simulink model "Dyn_Nonlinear_Forcefour"  (R2021a)
settings: Solver=VariableStepAuto  StartTime=0.0  StopTime=5  FixedStep=0.048  MaxStep=0.048  RelTol=1e-5
settings Model: Creator=zahra  LastModifiedBy=Dell 5520
settings SolverCC: AlgebraicLoopSolver=TrustRegion
settings DataIOCC: ReturnWorkspaceOutputs=off
settings DebuggingCC: ArithmeticOperatorsInVariantConditions=warning
settings SFSimCC: CustomCodeUndefinedFunction=UseInterfaceOnly
settings CodeAppCC: StateflowObjectComments=on

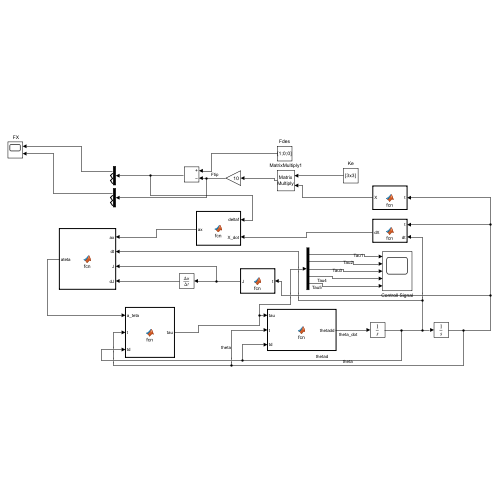
[thumbnail: Simulink's stored preview of the top-level diagram]
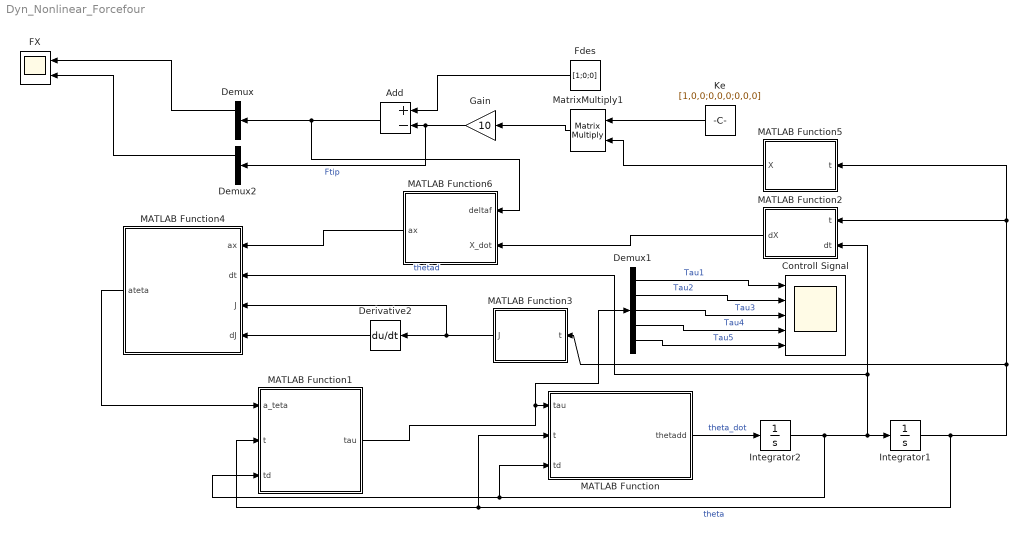
== system Dyn_Nonlinear_Forcefour ==
  " FX" : Scope  NumInputPorts=2
  Add : Sum  Inputs=+-
  Controll Signal : Scope  NumInputPorts=5
  Demux : Demux  Outputs=3
  Demux1 : Demux  Outputs=5
  Demux2 : Demux  Outputs=3
  Derivative2 : Derivative
  Fdes : Constant  Value=[1;0;0]
  Gain : Gain  Gain=10
  Integrator1 : Integrator  InitialCondition=[0;0;0;0;0]
  Integrator2 : Integrator  InitialCondition=[0;0;0;0;0]
  Ke : Constant  Value=[1,0,0;0,0,0;0,0,0]
  MATLAB Function : MATLAB Function  TreatAsAtomicUnit=on
  MATLAB Function1 : MATLAB Function  TreatAsAtomicUnit=on
  MATLAB Function2 : MATLAB Function  TreatAsAtomicUnit=on
  MATLAB Function3 : MATLAB Function  TreatAsAtomicUnit=on
  MATLAB Function4 : MATLAB Function  TreatAsAtomicUnit=on
  MATLAB Function5 : MATLAB Function  TreatAsAtomicUnit=on
  MATLAB Function6 : MATLAB Function  TreatAsAtomicUnit=on
  MatrixMultiply1 : Product  Multiplication=Matrix(*)
  wires:
  MATLAB Function/1(thetadd) -> Integrator2/1  "theta_dot"
  Integrator1/1 -> MATLAB Function5/1(t), MATLAB Function2/1(t), MATLAB Function3/1(t), MATLAB Function/2(t), MATLAB Function1/2(t)  "theta"
  Integrator2/1 -> MATLAB Function2/2(dt), MATLAB Function4/2(dt), Integrator1/1, MATLAB Function/3(td), MATLAB Function1/3(td)  "thetad"
  MATLAB Function1/1(tau) -> Demux1/1, MATLAB Function/1(tau)
  MATLAB Function3/1(J) -> MATLAB Function4/3(J), Derivative2/1
  Derivative2/1 -> MATLAB Function4/4(dJ)
  MATLAB Function6/1(ax) -> MATLAB Function4/1(ax)
  MATLAB Function4/1(ateta) -> MATLAB Function1/1(a_teta)
  MATLAB Function5/1(X) -> MatrixMultiply1/2
  MATLAB Function2/1(dX) -> MATLAB Function6/2(X_dot)
  Ke/1 -> MatrixMultiply1/1
  MatrixMultiply1/1 -> Gain/1
  Add/1 -> MATLAB Function6/1(deltaf), Demux/1
  Fdes/1 -> Add/1
  Demux/1 -> " FX"/1
  Gain/1 -> Demux2/1, Add/2  "Ftip"
  Demux1/4 -> Controll Signal/4  "Tau4"
  Demux1/5 -> Controll Signal/5  "Tau5"
  Demux1/1 -> Controll Signal/1  "Tau1"
  Demux1/2 -> Controll Signal/2  "Tau2"
  Demux1/3 -> Controll Signal/3  "Tau3"
  Demux2/1 -> " FX"/2

== matlab function Dyn_Nonlinear_Forcefour/MATLAB Function2 ==
  data: t input; dX output; dt input
function dX  = fcn(t,dt)
theta1 = t(1); theta2 = t(2); theta3 = t(3); 
theta4 = t(4); theta5 = t(5); 


T01 = [cos(theta1),0,sin(theta1),0;sin(theta1),0,-cos(theta1),0;0,1,0,0;0,0,0,1];
T12 = [cos(theta2),-sin(theta2),0,0.50*cos(theta2);sin(theta2),cos(theta2),0,0.50*sin(theta2);0,0,1,0;0,0,0,1];
T23 = [cos(theta3),-sin(theta3),0,0.50*cos(theta3);sin(theta3),cos(theta3),0,0.50*sin(theta3);0,0,1,0;0,0,0,1];
T34 = [cos(theta4),0,-sin(theta4),0;sin(theta4),0,cos(theta4),0;0,-1,0,0;0,0,0,1];
T45 = [cos(theta5),-sin(theta5),0,0;sin(theta5),cos(theta5),0,0;0,0,1,0.15;0,0,0,1];

T02 = T01 * T12 ;
T03 = T01 * T12 * T23 ; 
T04 = T01 * T12 * T23 * T34 ;
T0e=  T01 * T12 * T23 * T34 * T45 ;

z1 = T01(1:3, 3);
z2 = T02(1:3, 3);
z3 = T03(1:3, 3);
z4 = T04(1:3, 3);
z5 = T0e(1:3, 3);

o1 = T01(1:3, 4);
o2 = T02(1:3, 4);
o3 = T03(1:3, 4);
o4 = T04(1:3, 4);
o5 = T0e(1:3, 4);

J1 = [cross(z1, (o5 - o1))];
J2 = [cross(z2, (o5 - o2))];
J3 = [cross(z3, (o5 - o3))];
J4 = [cross(z4, (o5 - o4))];
J5 = [cross(z5, (o5 - o5))];
J_alternative_V = [J1 J2 J3 J4 J5];

J=J_alternative_V;

dX=J*dt;
return;

== matlab function Dyn_Nonlinear_Forcefour/MATLAB Function1 ==
  data: a_teta input; tau output; t input; td input
function tau  = fcn(a_teta, t, td)

theta1 = t(1); theta2 = t(2); theta3 = t(3); 
theta4 = t(4); theta5 = t(5);  

thetad1 = td(1); thetad2 = td(2); thetad3 = td(3);
thetad4 = td(4); thetad5 = td(5); 

M=zeros(5);
M(1,1) = 1.1807*cos(theta3) - 0.9672*cos(theta4) - 0.7031*sin(theta3) - 1.7889*sin(theta4) - 0.9672*cos(theta3)*cos(theta4) - 1.7889*cos(theta3)*sin(theta4) - 1.7889*cos(theta4)*sin(theta3) - 1.84*cos(theta5)*sin(theta5) + 0.9672*sin(theta3)*sin(theta4) - 1.17*cos(theta5)^2 + 11.017252 ;
M(1,2) = 0.59035*cos(theta3) - 0.9672*cos(theta4) - 0.35155*sin(theta3) - 1.7889*sin(theta4) - 0.4836*cos(theta3)*cos(theta4) - 0.89445*cos(theta3)*sin(theta4) - 0.89445*cos(theta4)*sin(theta3) - 1.84*cos(theta5)*sin(theta5) + 0.4836*sin(theta3)*sin(theta4) - 1.17*cos(theta5)^2 + 10.020592 ;
M(1,3) = 0.4836*sin(theta3)*sin(theta4) - 0.4836*cos(theta4) - 0.35155*sin(theta3) - 0.89445*sin(theta4) - 0.4836*cos(theta3)*cos(theta4) - 0.89445*cos(theta3)*sin(theta4) - 0.89445*cos(theta4)*sin(theta3) - 1.84*cos(theta5)*sin(theta5) - 0.16465*cos(theta3) - 1.17*cos(theta5)^2 + 9.175155 ;
M(1,4) = 0.98*sin(theta5) - 0.8928*sin(theta4) - 1.67*cos(theta5) - 0.8928*cos(theta3)*sin(theta4) - 0.8928*cos(theta4)*sin(theta3) + 0.008464 ;
M(1,5) = 0.98*sin(theta5) - 1.67*cos(theta5) ;
M(2,1) = 0.59035*cos(theta3) - 0.9672*cos(theta4) - 0.35155*sin(theta3) - 1.7889*sin(theta4) - 0.4836*cos(theta3)*cos(theta4) - 0.89445*cos(theta3)*sin(theta4) - 0.89445*cos(theta4)*sin(theta3) - 1.84*cos(theta5)*sin(theta5) + 0.4836*sin(theta3)*sin(theta4) - 1.17*cos(theta5)^2 + 10.020592 ;
M(2,2) = 10.133642 - 1.7889*sin(theta4) - 1.84*cos(theta5)*sin(theta5) - 1.17*cos(theta5)^2 - 0.9672*cos(theta4) ;
M(2,3) = 9.175155 - 0.89445*sin(theta4) - 1.84*cos(theta5)*sin(theta5) - 1.17*cos(theta5)^2 - 0.4836*cos(theta4) ;
M(2,4) = 0.98*sin(theta5) - 0.8928*sin(theta4) - 1.67*cos(theta5) + 0.008464 ;
M(2,5) = 0.98*sin(theta5) - 1.67*cos(theta5) ;
M(3,1) = 0.4836*sin(theta3)*sin(theta4) - 0.4836*cos(theta4) - 0.35155*sin(theta3) - 0.89445*sin(theta4) - 0.4836*cos(theta3)*cos(theta4) - 0.89445*cos(theta3)*sin(theta4) - 0.89445*cos(theta4)*sin(theta3) - 1.84*cos(theta5)*sin(theta5) - 0.16465*cos(theta3) - 1.17*cos(theta5)^2 + 9.175155 ;
M(3,2) = 9.175155 - 0.89445*sin(theta4) - 1.84*cos(theta5)*sin(theta5) - 1.17*cos(theta5)^2 - 0.4836*cos(theta4) ;
M(3,3) = 9.339805 - 1.17*cos(theta5)^2 - 1.84*cos(theta5)*sin(theta5) ;
M(3,4) = 0.98*sin(theta5) - 1.67*cos(theta5) + 0.008464 ;
M(3,5) = 0.98*sin(theta5) - 1.67*cos(theta5) ;
M(4,1) = 0.98*sin(theta5) - 0.8928*sin(theta4) - 1.67*cos(theta5) - 0.8928*cos(theta3)*sin(theta4) - 0.8928*cos(theta4)*sin(theta3) + 0.008464 ;
M(4,2) = 0.98*sin(theta5) - 0.8928*sin(theta4) - 1.67*cos(theta5) + 0.008464 ;
M(4,3) = 0.98*sin(theta5) - 1.67*cos(theta5) + 0.008464 ;
M(4,4) = 6.81712 ;
M(4,5) = 2.3 ;
M(5,1) = 0.98*sin(theta5) - 1.67*cos(theta5) ;
M(5,2) = 0.98*sin(theta5) - 1.67*cos(theta5) ;
M(5,3) = 0.98*sin(theta5) - 1.67*cos(theta5) ;
M(5,4) = 2.3 ;
M(5,5) = 2.3 ;


C=zeros(5);
C(1,1) = 0.92*thetad5 - 1.84*thetad5*cos(theta5)^2 - 0.35155*thetad3*cos(theta3) - 0.89445*thetad4*cos(theta4) - 0.59035*thetad3*sin(theta3) + 0.4836*thetad4*sin(theta4) - 0.89445*thetad3*cos(theta3)*cos(theta4) - 0.89445*thetad4*cos(theta3)*cos(theta4) + 0.4836*thetad3*cos(theta3)*sin(theta4) + 0.4836*thetad3*cos(theta4)*sin(theta3) + 0.4836*thetad4*cos(theta3)*sin(theta4) + 0.4836*thetad4*cos(theta4)*sin(theta3) + 1.17*thetad5*cos(theta5)*sin(theta5) + 0.89445*thetad3*sin(theta3)*sin(theta4) + 0.89445*thetad4*sin(theta3)*sin(theta4) ;
C(1,2) = 0.92*thetad5 - 1.84*thetad5*cos(theta5)^2 - 0.175775*thetad3*cos(theta3) - 0.89445*thetad4*cos(theta4) - 0.295175*thetad3*sin(theta3) + 0.4836*thetad4*sin(theta4) - 0.447225*thetad3*cos(theta3)*cos(theta4) - 0.447225*thetad4*cos(theta3)*cos(theta4) + 0.2418*thetad3*cos(theta3)*sin(theta4) + 0.2418*thetad3*cos(theta4)*sin(theta3) + 0.2418*thetad4*cos(theta3)*sin(theta4) + 0.2418*thetad4*cos(theta4)*sin(theta3) + 1.17*thetad5*cos(theta5)*sin(theta5) + 0.447225*thetad3*sin(theta3)*sin(theta4) + 0.447225*thetad4*sin(theta3)*sin(theta4) ;
C(1,3) = 0.92*thetad5 - 1.84*thetad5*cos(theta5)^2 - 0.35155*thetad1*cos(theta3) - 0.175775*thetad2*cos(theta3) - 0.35155*thetad3*cos(theta3) - 0.447225*thetad4*cos(theta4) - 0.59035*thetad1*sin(theta3) - 0.295175*thetad2*sin(theta3) + 0.16465*thetad3*sin(theta3) + 0.2418*thetad4*sin(theta4) - 0.89445*thetad1*cos(theta3)*cos(theta4) - 0.447225*thetad2*cos(theta3)*cos(theta4) - 0.89445*thetad3*cos(theta3)*cos(theta4) - 0.893625*thetad4*cos(theta3)*cos(theta4) + 0.4836*thetad1*cos(theta3)*sin(theta4) + 0.4836*thetad1*cos(theta4)*sin(theta3) + 0.2418*thetad2*cos(theta3)*sin(theta4) + 0.2418*thetad2*cos(theta4)*sin(theta3) + 0.4836*thetad3*cos(theta3)*sin(theta4) + 0.4836*thetad3*cos(theta4)*sin(theta3) + 0.2418*thetad4*cos(theta3)*sin(theta4) + 0.2418*thetad4*cos(theta4)*sin(theta3) + 1.17*thetad5*cos(theta5)*sin(theta5) + 0.89445*thetad1*sin(theta3)*sin(theta4) + 0.447225*thetad2*sin(theta3)*sin(theta4) + 0.89445*thetad3*sin(theta3)*sin(theta4) + 0.893625*thetad4*sin(theta3)*sin(theta4) ;
C(1,4) = 0.49*thetad5*cos(theta5) - 0.89445*thetad2*cos(theta4) - 0.447225*thetad3*cos(theta4) - 0.8928*thetad4*cos(theta4) - 0.89445*thetad1*cos(theta4) + 0.4836*thetad1*sin(theta4) + 0.4836*thetad2*sin(theta4) + 0.2418*thetad3*sin(theta4) + 0.835*thetad5*sin(theta5) - 0.89445*thetad1*cos(theta3)*cos(theta4) - 0.447225*thetad2*cos(theta3)*cos(theta4) - 0.893625*thetad3*cos(theta3)*cos(theta4) - 0.8928*thetad4*cos(theta3)*cos(theta4) + 0.4836*thetad1*cos(theta3)*sin(theta4) + 0.4836*thetad1*cos(theta4)*sin(theta3) + 0.2418*thetad2*cos(theta3)*sin(theta4) + 0.2418*thetad2*cos(theta4)*sin(theta3) + 0.2418*thetad3*cos(theta3)*sin(theta4) + 0.2418*thetad3*cos(theta4)*sin(theta3) + 0.89445*thetad1*sin(theta3)*sin(theta4) + 0.447225*thetad2*sin(theta3)*sin(theta4) + 0.893625*thetad3*sin(theta3)*sin(theta4) + 0.8928*thetad4*sin(theta3)*sin(theta4) ;
C(1,5) = 0.92*thetad1 + 0.92*thetad2 + 0.92*thetad3 - 1.84*thetad1*cos(theta5)^2 - 1.84*thetad2*cos(theta5)^2 - 1.84*thetad3*cos(theta5)^2 + 0.49*thetad4*cos(theta5) + 0.98*thetad5*cos(theta5) + 0.835*thetad4*sin(theta5) + 1.67*thetad5*sin(theta5) + 1.17*thetad1*cos(theta5)*sin(theta5) + 1.17*thetad2*cos(theta5)*sin(theta5) + 1.17*thetad3*cos(theta5)*sin(theta5) ;
C(2,1) = 0.92*thetad5 - 1.84*thetad5*cos(theta5)^2 - 0.175775*thetad3*cos(theta3) - 0.89445*thetad4*cos(theta4) - 0.295175*thetad3*sin(theta3) + 0.4836*thetad4*sin(theta4) - 0.447225*thetad3*cos(theta3)*cos(theta4) - 0.447225*thetad4*cos(theta3)*cos(theta4) + 0.2418*thetad3*cos(theta3)*sin(theta4) + 0.2418*thetad3*cos(theta4)*sin(theta3) + 0.2418*thetad4*cos(theta3)*sin(theta4) + 0.2418*thetad4*cos(theta4)*sin(theta3) + 1.17*thetad5*cos(theta5)*sin(theta5) + 0.447225*thetad3*sin(theta3)*sin(theta4) + 0.447225*thetad4*sin(theta3)*sin(theta4) ;
C(2,2) = 0.92*thetad5 - 1.84*thetad5*cos(theta5)^2 - 0.89445*thetad4*cos(theta4) + 0.4836*thetad4*sin(theta4) + 1.17*thetad5*cos(theta5)*sin(theta5) ;
C(2,3) = 0.92*thetad5 - 1.84*thetad5*cos(theta5)^2 - 0.175775*thetad1*cos(theta3) - 0.447225*thetad4*cos(theta4) - 0.295175*thetad1*sin(theta3) + 0.2418*thetad4*sin(theta4) - 0.447225*thetad1*cos(theta3)*cos(theta4) + 0.2418*thetad1*cos(theta3)*sin(theta4) + 0.2418*thetad1*cos(theta4)*sin(theta3) + 1.17*thetad5*cos(theta5)*sin(theta5) + 0.447225*thetad1*sin(theta3)*sin(theta4) ;
C(2,4) = 0.49*thetad5*cos(theta5) - 0.89445*thetad2*cos(theta4) - 0.447225*thetad3*cos(theta4) - 0.8928*thetad4*cos(theta4) - 0.89445*thetad1*cos(theta4) + 0.4836*thetad1*sin(theta4) + 0.4836*thetad2*sin(theta4) + 0.2418*thetad3*sin(theta4) + 0.835*thetad5*sin(theta5) - 0.447225*thetad1*cos(theta3)*cos(theta4) + 0.2418*thetad1*cos(theta3)*sin(theta4) + 0.2418*thetad1*cos(theta4)*sin(theta3) + 0.447225*thetad1*sin(theta3)*sin(theta4) ;
C(2,5) = 0.92*thetad1 + 0.92*thetad2 + 0.92*thetad3 - 1.84*thetad1*cos(theta5)^2 - 1.84*thetad2*cos(theta5)^2 - 1.84*thetad3*cos(theta5)^2 + 0.49*thetad4*cos(theta5) + 0.98*thetad5*cos(theta5) + 0.835*thetad4*sin(theta5) + 1.67*thetad5*sin(theta5) + 1.17*thetad1*cos(theta5)*sin(theta5) + 1.17*thetad2*cos(theta5)*sin(theta5) + 1.17*thetad3*cos(theta5)*sin(theta5) ;
C(3,1) = 0.92*thetad5 - 1.84*thetad5*cos(theta5)^2 + 0.35155*thetad1*cos(theta3) + 0.175775*thetad2*cos(theta3) - 0.447225*thetad4*cos(theta4) + 0.59035*thetad1*sin(theta3) + 0.295175*thetad2*sin(theta3) + 0.2418*thetad4*sin(theta4) + 0.89445*thetad1*cos(theta3)*cos(theta4) + 0.447225*thetad2*cos(theta3)*cos(theta4) - 0.000825*thetad4*cos(theta3)*cos(theta4) - 0.4836*thetad1*cos(theta3)*sin(theta4) - 0.4836*thetad1*cos(theta4)*sin(theta3) - 0.2418*thetad2*cos(theta3)*sin(theta4) - 0.2418*thetad2*cos(theta4)*sin(theta3) + 0.2418*thetad4*cos(theta3)*sin(theta4) + 0.2418*thetad4*cos(theta4)*sin(theta3) + 1.17*thetad5*cos(theta5)*sin(theta5) - 0.89445*thetad1*sin(theta3)*sin(theta4) - 0.447225*thetad2*sin(theta3)*sin(theta4) + 0.000825*thetad4*sin(theta3)*sin(theta4) ;
C(3,2) = 0.92*thetad5 - 1.84*thetad5*cos(theta5)^2 + 0.175775*thetad1*cos(theta3) - 0.447225*thetad4*cos(theta4) + 0.295175*thetad1*sin(theta3) + 0.2418*thetad4*sin(theta4) + 0.447225*thetad1*cos(theta3)*cos(theta4) - 0.2418*thetad1*cos(theta3)*sin(theta4) - 0.2418*thetad1*cos(theta4)*sin(theta3) + 1.17*thetad5*cos(theta5)*sin(theta5) - 0.447225*thetad1*sin(theta3)*sin(theta4) ;
C(3,3) = 0.92*thetad5 - 1.84*thetad5*cos(theta5)^2 + 1.17*thetad5*cos(theta5)*sin(theta5) ;
C(3,4) = 0.49*thetad5*cos(theta5) - 0.447225*thetad2*cos(theta4) - 0.447225*thetad1*cos(theta4) + 0.2418*thetad1*sin(theta4) + 0.2418*thetad2*sin(theta4) + 0.835*thetad5*sin(theta5) - 0.000825*thetad1*cos(theta3)*cos(theta4) + 0.2418*thetad1*cos(theta3)*sin(theta4) + 0.2418*thetad1*cos(theta4)*sin(theta3) + 0.000825*thetad1*sin(theta3)*sin(theta4) ;
C(3,5) = 0.92*thetad1 + 0.92*thetad2 + 0.92*thetad3 - 1.84*thetad1*cos(theta5)^2 - 1.84*thetad2*cos(theta5)^2 - 1.84*thetad3*cos(theta5)^2 + 0.49*thetad4*cos(theta5) + 0.98*thetad5*cos(theta5) + 0.835*thetad4*sin(theta5) + 1.67*thetad5*sin(theta5) + 1.17*thetad1*cos(theta5)*sin(theta5) + 1.17*thetad2*cos(theta5)*sin(theta5) + 1.17*thetad3*cos(theta5)*sin(theta5) ;
C(4,1) = 0.89445*thetad1*cos(theta4) + 0.89445*thetad2*cos(theta4) + 0.447225*thetad3*cos(theta4) + 0.49*thetad5*cos(theta5) - 0.4836*thetad1*sin(theta4) - 0.4836*thetad2*sin(theta4) - 0.2418*thetad3*sin(theta4) + 0.835*thetad5*sin(theta5) + 0.89445*thetad1*cos(theta3)*cos(theta4) + 0.447225*thetad2*cos(theta3)*cos(theta4) + 0.000825*thetad3*cos(theta3)*cos(theta4) - 0.4836*thetad1*cos(theta3)*sin(theta4) - 0.4836*thetad1*cos(theta4)*sin(theta3) - 0.2418*thetad2*cos(theta3)*sin(theta4) - 0.2418*thetad2*cos(theta4)*sin(theta3) - 0.2418*thetad3*cos(theta3)*sin(theta4) - 0.2418*thetad3*cos(theta4)*sin(theta3) - 0.89445*thetad1*sin(theta3)*sin(theta4) - 0.447225*thetad2*sin(theta3)*sin(theta4) - 0.000825*thetad3*sin(theta3)*sin(theta4) ;
C(4,2) = 0.89445*thetad1*cos(theta4) + 0.89445*thetad2*cos(theta4) + 0.447225*thetad3*cos(theta4) + 0.49*thetad5*cos(theta5) - 0.4836*thetad1*sin(theta4) - 0.4836*thetad2*sin(theta4) - 0.2418*thetad3*sin(theta4) + 0.835*thetad5*sin(theta5) + 0.447225*thetad1*cos(theta3)*cos(theta4) - 0.2418*thetad1*cos(theta3)*sin(theta4) - 0.2418*thetad1*cos(theta4)*sin(theta3) - 0.447225*thetad1*sin(theta3)*sin(theta4) ;
C(4,3) = 0.447225*thetad1*cos(theta4) + 0.447225*thetad2*cos(theta4) + 0.49*thetad5*cos(theta5) - 0.2418*thetad1*sin(theta4) - 0.2418*thetad2*sin(theta4) + 0.835*thetad5*sin(theta5) + 0.000825*thetad1*cos(theta3)*cos(theta4) - 0.2418*thetad1*cos(theta3)*sin(theta4) - 0.2418*thetad1*cos(theta4)*sin(theta3) - 0.000825*thetad1*sin(theta3)*sin(theta4) ;
C(4,4) = 0.0 ;
C(4,5) = 0.49*thetad1*cos(theta5) + 0.49*thetad2*cos(theta5) + 0.49*thetad3*cos(theta5) + 0.835*thetad1*sin(theta5) + 0.835*thetad2*sin(theta5) + 0.835*thetad3*sin(theta5) ;
C(5,1) = 1.84*thetad1*cos(theta5)^2 - 0.92*thetad2 - 0.92*thetad3 - 0.92*thetad1 + 1.84*thetad2*cos(theta5)^2 + 1.84*thetad3*cos(theta5)^2 - 0.49*thetad4*cos(theta5) - 0.835*thetad4*sin(theta5) - 1.17*thetad1*cos(theta5)*sin(theta5) - 1.17*thetad2*cos(theta5)*sin(theta5) - 1.17*thetad3*cos(theta5)*sin(theta5) ;
C(5,2) = 1.84*thetad1*cos(theta5)^2 - 0.92*thetad2 - 0.92*thetad3 - 0.92*thetad1 + 1.84*thetad2*cos(theta5)^2 + 1.84*thetad3*cos(theta5)^2 - 0.49*thetad4*cos(theta5) - 0.835*thetad4*sin(theta5) - 1.17*thetad1*cos(theta5)*sin(theta5) - 1.17*thetad2*cos(theta5)*sin(theta5) - 1.17*thetad3*cos(theta5)*sin(theta5) ;
C(5,3) = 1.84*thetad1*cos(theta5)^2 - 0.92*thetad2 - 0.92*thetad3 - 0.92*thetad1 + 1.84*thetad2*cos(theta5)^2 + 1.84*thetad3*cos(theta5)^2 - 0.49*thetad4*cos(theta5) - 0.835*thetad4*sin(theta5) - 1.17*thetad1*cos(theta5)*sin(theta5) - 1.17*thetad2*cos(theta5)*sin(theta5) - 1.17*thetad3*cos(theta5)*sin(theta5) ;
C(5,4) = - 0.49*thetad1*cos(theta5) - 0.49*thetad2*cos(theta5) - 0.49*thetad3*cos(theta5) - 0.835*thetad1*sin(theta5) - 0.835*thetad2*sin(theta5) - 0.835*thetad3*sin(theta5) ;
C(5,5) = 0.0 ;



G=zeros(5,1);
G(1) = 0.0 ;
G(2) = 19.118709000000000552432766198763*cos(theta2) - 3.9141900000000005022116056352388*sin(theta2) + 11.582667*cos(theta2)*cos(theta3) - 6.897411*cos(theta2)*sin(theta3) - 6.897411*cos(theta3)*sin(theta2) - 11.582667*sin(theta2)*sin(theta3) + 9.488232*cos(theta2)*sin(theta3)*sin(theta4) + 9.488232*cos(theta3)*sin(theta2)*sin(theta4) + 9.488232*cos(theta4)*sin(theta2)*sin(theta3) + 17.549109*sin(theta2)*sin(theta3)*sin(theta4) - 9.488232*cos(theta2)*cos(theta3)*cos(theta4) - 17.549109*cos(theta2)*cos(theta3)*sin(theta4) - 17.549109*cos(theta2)*cos(theta4)*sin(theta3) - 17.549109*cos(theta3)*cos(theta4)*sin(theta2) ;
G(3) = 11.582667*cos(theta2)*cos(theta3) - 6.897411*cos(theta2)*sin(theta3) - 6.897411*cos(theta3)*sin(theta2) - 11.582667*sin(theta2)*sin(theta3) + 9.488232*cos(theta2)*sin(theta3)*sin(theta4) + 9.488232*cos(theta3)*sin(theta2)*sin(theta4) + 9.488232*cos(theta4)*sin(theta2)*sin(theta3) + 17.549109*sin(theta2)*sin(theta3)*sin(theta4) - 9.488232*cos(theta2)*cos(theta3)*cos(theta4) - 17.549109*cos(theta2)*cos(theta3)*sin(theta4) - 17.549109*cos(theta2)*cos(theta4)*sin(theta3) - 17.549109*cos(theta3)*cos(theta4)*sin(theta2) ;
G(4) = 9.488232*cos(theta2)*sin(theta3)*sin(theta4) + 9.488232*cos(theta3)*sin(theta2)*sin(theta4) + 9.488232*cos(theta4)*sin(theta2)*sin(theta3) + 17.549109*sin(theta2)*sin(theta3)*sin(theta4) - 9.488232*cos(theta2)*cos(theta3)*cos(theta4) - 17.549109*cos(theta2)*cos(theta3)*sin(theta4) - 17.549109*cos(theta2)*cos(theta4)*sin(theta3) - 17.549109*cos(theta3)*cos(theta4)*sin(theta2) ;
G(5) = 0.0 ;


tau = M*a_teta+C*td+G;


return

== matlab function Dyn_Nonlinear_Forcefour/MATLAB Function ==
  data: thetadd output; tau input; t input; td input
function thetadd  = fcn(tau, t, td)
theta1 = t(1); theta2 = t(2); theta3 = t(3); 
theta4 = t(4); theta5 = t(5);  

thetad1 = td(1); thetad2 = td(2); thetad3 = td(3);
thetad4 = td(4); thetad5 = td(5); 

M=zeros(5);
M(1,1) = 1.1807*cos(theta3) - 0.9672*cos(theta4) - 0.7031*sin(theta3) - 1.7889*sin(theta4) - 0.9672*cos(theta3)*cos(theta4) - 1.7889*cos(theta3)*sin(theta4) - 1.7889*cos(theta4)*sin(theta3) - 1.84*cos(theta5)*sin(theta5) + 0.9672*sin(theta3)*sin(theta4) - 1.17*cos(theta5)^2 + 11.017252 ;
M(1,2) = 0.59035*cos(theta3) - 0.9672*cos(theta4) - 0.35155*sin(theta3) - 1.7889*sin(theta4) - 0.4836*cos(theta3)*cos(theta4) - 0.89445*cos(theta3)*sin(theta4) - 0.89445*cos(theta4)*sin(theta3) - 1.84*cos(theta5)*sin(theta5) + 0.4836*sin(theta3)*sin(theta4) - 1.17*cos(theta5)^2 + 10.020592 ;
M(1,3) = 0.4836*sin(theta3)*sin(theta4) - 0.4836*cos(theta4) - 0.35155*sin(theta3) - 0.89445*sin(theta4) - 0.4836*cos(theta3)*cos(theta4) - 0.89445*cos(theta3)*sin(theta4) - 0.89445*cos(theta4)*sin(theta3) - 1.84*cos(theta5)*sin(theta5) - 0.16465*cos(theta3) - 1.17*cos(theta5)^2 + 9.175155 ;
M(1,4) = 0.98*sin(theta5) - 0.8928*sin(theta4) - 1.67*cos(theta5) - 0.8928*cos(theta3)*sin(theta4) - 0.8928*cos(theta4)*sin(theta3) + 0.008464 ;
M(1,5) = 0.98*sin(theta5) - 1.67*cos(theta5) ;
M(2,1) = 0.59035*cos(theta3) - 0.9672*cos(theta4) - 0.35155*sin(theta3) - 1.7889*sin(theta4) - 0.4836*cos(theta3)*cos(theta4) - 0.89445*cos(theta3)*sin(theta4) - 0.89445*cos(theta4)*sin(theta3) - 1.84*cos(theta5)*sin(theta5) + 0.4836*sin(theta3)*sin(theta4) - 1.17*cos(theta5)^2 + 10.020592 ;
M(2,2) = 10.133642 - 1.7889*sin(theta4) - 1.84*cos(theta5)*sin(theta5) - 1.17*cos(theta5)^2 - 0.9672*cos(theta4) ;
M(2,3) = 9.175155 - 0.89445*sin(theta4) - 1.84*cos(theta5)*sin(theta5) - 1.17*cos(theta5)^2 - 0.4836*cos(theta4) ;
M(2,4) = 0.98*sin(theta5) - 0.8928*sin(theta4) - 1.67*cos(theta5) + 0.008464 ;
M(2,5) = 0.98*sin(theta5) - 1.67*cos(theta5) ;
M(3,1) = 0.4836*sin(theta3)*sin(theta4) - 0.4836*cos(theta4) - 0.35155*sin(theta3) - 0.89445*sin(theta4) - 0.4836*cos(theta3)*cos(theta4) - 0.89445*cos(theta3)*sin(theta4) - 0.89445*cos(theta4)*sin(theta3) - 1.84*cos(theta5)*sin(theta5) - 0.16465*cos(theta3) - 1.17*cos(theta5)^2 + 9.175155 ;
M(3,2) = 9.175155 - 0.89445*sin(theta4) - 1.84*cos(theta5)*sin(theta5) - 1.17*cos(theta5)^2 - 0.4836*cos(theta4) ;
M(3,3) = 9.339805 - 1.17*cos(theta5)^2 - 1.84*cos(theta5)*sin(theta5) ;
M(3,4) = 0.98*sin(theta5) - 1.67*cos(theta5) + 0.008464 ;
M(3,5) = 0.98*sin(theta5) - 1.67*cos(theta5) ;
M(4,1) = 0.98*sin(theta5) - 0.8928*sin(theta4) - 1.67*cos(theta5) - 0.8928*cos(theta3)*sin(theta4) - 0.8928*cos(theta4)*sin(theta3) + 0.008464 ;
M(4,2) = 0.98*sin(theta5) - 0.8928*sin(theta4) - 1.67*cos(theta5) + 0.008464 ;
M(4,3) = 0.98*sin(theta5) - 1.67*cos(theta5) + 0.008464 ;
M(4,4) = 6.81712 ;
M(4,5) = 2.3 ;
M(5,1) = 0.98*sin(theta5) - 1.67*cos(theta5) ;
M(5,2) = 0.98*sin(theta5) - 1.67*cos(theta5) ;
M(5,3) = 0.98*sin(theta5) - 1.67*cos(theta5) ;
M(5,4) = 2.3 ;
M(5,5) = 2.3 ;


C=zeros(5);
C(1,1) = 0.92*thetad5 - 1.84*thetad5*cos(theta5)^2 - 0.35155*thetad3*cos(theta3) - 0.89445*thetad4*cos(theta4) - 0.59035*thetad3*sin(theta3) + 0.4836*thetad4*sin(theta4) - 0.89445*thetad3*cos(theta3)*cos(theta4) - 0.89445*thetad4*cos(theta3)*cos(theta4) + 0.4836*thetad3*cos(theta3)*sin(theta4) + 0.4836*thetad3*cos(theta4)*sin(theta3) + 0.4836*thetad4*cos(theta3)*sin(theta4) + 0.4836*thetad4*cos(theta4)*sin(theta3) + 1.17*thetad5*cos(theta5)*sin(theta5) + 0.89445*thetad3*sin(theta3)*sin(theta4) + 0.89445*thetad4*sin(theta3)*sin(theta4) ;
C(1,2) = 0.92*thetad5 - 1.84*thetad5*cos(theta5)^2 - 0.175775*thetad3*cos(theta3) - 0.89445*thetad4*cos(theta4) - 0.295175*thetad3*sin(theta3) + 0.4836*thetad4*sin(theta4) - 0.447225*thetad3*cos(theta3)*cos(theta4) - 0.447225*thetad4*cos(theta3)*cos(theta4) + 0.2418*thetad3*cos(theta3)*sin(theta4) + 0.2418*thetad3*cos(theta4)*sin(theta3) + 0.2418*thetad4*cos(theta3)*sin(theta4) + 0.2418*thetad4*cos(theta4)*sin(theta3) + 1.17*thetad5*cos(theta5)*sin(theta5) + 0.447225*thetad3*sin(theta3)*sin(theta4) + 0.447225*thetad4*sin(theta3)*sin(theta4) ;
C(1,3) = 0.92*thetad5 - 1.84*thetad5*cos(theta5)^2 - 0.35155*thetad1*cos(theta3) - 0.175775*thetad2*cos(theta3) - 0.35155*thetad3*cos(theta3) - 0.447225*thetad4*cos(theta4) - 0.59035*thetad1*sin(theta3) - 0.295175*thetad2*sin(theta3) + 0.16465*thetad3*sin(theta3) + 0.2418*thetad4*sin(theta4) - 0.89445*thetad1*cos(theta3)*cos(theta4) - 0.447225*thetad2*cos(theta3)*cos(theta4) - 0.89445*thetad3*cos(theta3)*cos(theta4) - 0.893625*thetad4*cos(theta3)*cos(theta4) + 0.4836*thetad1*cos(theta3)*sin(theta4) + 0.4836*thetad1*cos(theta4)*sin(theta3) + 0.2418*thetad2*cos(theta3)*sin(theta4) + 0.2418*thetad2*cos(theta4)*sin(theta3) + 0.4836*thetad3*cos(theta3)*sin(theta4) + 0.4836*thetad3*cos(theta4)*sin(theta3) + 0.2418*thetad4*cos(theta3)*sin(theta4) + 0.2418*thetad4*cos(theta4)*sin(theta3) + 1.17*thetad5*cos(theta5)*sin(theta5) + 0.89445*thetad1*sin(theta3)*sin(theta4) + 0.447225*thetad2*sin(theta3)*sin(theta4) + 0.89445*thetad3*sin(theta3)*sin(theta4) + 0.893625*thetad4*sin(theta3)*sin(theta4) ;
C(1,4) = 0.49*thetad5*cos(theta5) - 0.89445*thetad2*cos(theta4) - 0.447225*thetad3*cos(theta4) - 0.8928*thetad4*cos(theta4) - 0.89445*thetad1*cos(theta4) + 0.4836*thetad1*sin(theta4) + 0.4836*thetad2*sin(theta4) + 0.2418*thetad3*sin(theta4) + 0.835*thetad5*sin(theta5) - 0.89445*thetad1*cos(theta3)*cos(theta4) - 0.447225*thetad2*cos(theta3)*cos(theta4) - 0.893625*thetad3*cos(theta3)*cos(theta4) - 0.8928*thetad4*cos(theta3)*cos(theta4) + 0.4836*thetad1*cos(theta3)*sin(theta4) + 0.4836*thetad1*cos(theta4)*sin(theta3) + 0.2418*thetad2*cos(theta3)*sin(theta4) + 0.2418*thetad2*cos(theta4)*sin(theta3) + 0.2418*thetad3*cos(theta3)*sin(theta4) + 0.2418*thetad3*cos(theta4)*sin(theta3) + 0.89445*thetad1*sin(theta3)*sin(theta4) + 0.447225*thetad2*sin(theta3)*sin(theta4) + 0.893625*thetad3*sin(theta3)*sin(theta4) + 0.8928*thetad4*sin(theta3)*sin(theta4) ;
C(1,5) = 0.92*thetad1 + 0.92*thetad2 + 0.92*thetad3 - 1.84*thetad1*cos(theta5)^2 - 1.84*thetad2*cos(theta5)^2 - 1.84*thetad3*cos(theta5)^2 + 0.49*thetad4*cos(theta5) + 0.98*thetad5*cos(theta5) + 0.835*thetad4*sin(theta5) + 1.67*thetad5*sin(theta5) + 1.17*thetad1*cos(theta5)*sin(theta5) + 1.17*thetad2*cos(theta5)*sin(theta5) + 1.17*thetad3*cos(theta5)*sin(theta5) ;
C(2,1) = 0.92*thetad5 - 1.84*thetad5*cos(theta5)^2 - 0.175775*thetad3*cos(theta3) - 0.89445*thetad4*cos(theta4) - 0.295175*thetad3*sin(theta3) + 0.4836*thetad4*sin(theta4) - 0.447225*thetad3*cos(theta3)*cos(theta4) - 0.447225*thetad4*cos(theta3)*cos(theta4) + 0.2418*thetad3*cos(theta3)*sin(theta4) + 0.2418*thetad3*cos(theta4)*sin(theta3) + 0.2418*thetad4*cos(theta3)*sin(theta4) + 0.2418*thetad4*cos(theta4)*sin(theta3) + 1.17*thetad5*cos(theta5)*sin(theta5) + 0.447225*thetad3*sin(theta3)*sin(theta4) + 0.447225*thetad4*sin(theta3)*sin(theta4) ;
C(2,2) = 0.92*thetad5 - 1.84*thetad5*cos(theta5)^2 - 0.89445*thetad4*cos(theta4) + 0.4836*thetad4*sin(theta4) + 1.17*thetad5*cos(theta5)*sin(theta5) ;
C(2,3) = 0.92*thetad5 - 1.84*thetad5*cos(theta5)^2 - 0.175775*thetad1*cos(theta3) - 0.447225*thetad4*cos(theta4) - 0.295175*thetad1*sin(theta3) + 0.2418*thetad4*sin(theta4) - 0.447225*thetad1*cos(theta3)*cos(theta4) + 0.2418*thetad1*cos(theta3)*sin(theta4) + 0.2418*thetad1*cos(theta4)*sin(theta3) + 1.17*thetad5*cos(theta5)*sin(theta5) + 0.447225*thetad1*sin(theta3)*sin(theta4) ;
C(2,4) = 0.49*thetad5*cos(theta5) - 0.89445*thetad2*cos(theta4) - 0.447225*thetad3*cos(theta4) - 0.8928*thetad4*cos(theta4) - 0.89445*thetad1*cos(theta4) + 0.4836*thetad1*sin(theta4) + 0.4836*thetad2*sin(theta4) + 0.2418*thetad3*sin(theta4) + 0.835*thetad5*sin(theta5) - 0.447225*thetad1*cos(theta3)*cos(theta4) + 0.2418*thetad1*cos(theta3)*sin(theta4) + 0.2418*thetad1*cos(theta4)*sin(theta3) + 0.447225*thetad1*sin(theta3)*sin(theta4) ;
C(2,5) = 0.92*thetad1 + 0.92*thetad2 + 0.92*thetad3 - 1.84*thetad1*cos(theta5)^2 - 1.84*thetad2*cos(theta5)^2 - 1.84*thetad3*cos(theta5)^2 + 0.49*thetad4*cos(theta5) + 0.98*thetad5*cos(theta5) + 0.835*thetad4*sin(theta5) + 1.67*thetad5*sin(theta5) + 1.17*thetad1*cos(theta5)*sin(theta5) + 1.17*thetad2*cos(theta5)*sin(theta5) + 1.17*thetad3*cos(theta5)*sin(theta5) ;
C(3,1) = 0.92*thetad5 - 1.84*thetad5*cos(theta5)^2 + 0.35155*thetad1*cos(theta3) + 0.175775*thetad2*cos(theta3) - 0.447225*thetad4*cos(theta4) + 0.59035*thetad1*sin(theta3) + 0.295175*thetad2*sin(theta3) + 0.2418*thetad4*sin(theta4) + 0.89445*thetad1*cos(theta3)*cos(theta4) + 0.447225*thetad2*cos(theta3)*cos(theta4) - 0.000825*thetad4*cos(theta3)*cos(theta4) - 0.4836*thetad1*cos(theta3)*sin(theta4) - 0.4836*thetad1*cos(theta4)*sin(theta3) - 0.2418*thetad2*cos(theta3)*sin(theta4) - 0.2418*thetad2*cos(theta4)*sin(theta3) + 0.2418*thetad4*cos(theta3)*sin(theta4) + 0.2418*thetad4*cos(theta4)*sin(theta3) + 1.17*thetad5*cos(theta5)*sin(theta5) - 0.89445*thetad1*sin(theta3)*sin(theta4) - 0.447225*thetad2*sin(theta3)*sin(theta4) + 0.000825*thetad4*sin(theta3)*sin(theta4) ;
C(3,2) = 0.92*thetad5 - 1.84*thetad5*cos(theta5)^2 + 0.175775*thetad1*cos(theta3) - 0.447225*thetad4*cos(theta4) + 0.295175*thetad1*sin(theta3) + 0.2418*thetad4*sin(theta4) + 0.447225*thetad1*cos(theta3)*cos(theta4) - 0.2418*thetad1*cos(theta3)*sin(theta4) - 0.2418*thetad1*cos(theta4)*sin(theta3) + 1.17*thetad5*cos(theta5)*sin(theta5) - 0.447225*thetad1*sin(theta3)*sin(theta4) ;
C(3,3) = 0.92*thetad5 - 1.84*thetad5*cos(theta5)^2 + 1.17*thetad5*cos(theta5)*sin(theta5) ;
C(3,4) = 0.49*thetad5*cos(theta5) - 0.447225*thetad2*cos(theta4) - 0.447225*thetad1*cos(theta4) + 0.2418*thetad1*sin(theta4) + 0.2418*thetad2*sin(theta4) + 0.835*thetad5*sin(theta5) - 0.000825*thetad1*cos(theta3)*cos(theta4) + 0.2418*thetad1*cos(theta3)*sin(theta4) + 0.2418*thetad1*cos(theta4)*sin(theta3) + 0.000825*thetad1*sin(theta3)*sin(theta4) ;
C(3,5) = 0.92*thetad1 + 0.92*thetad2 + 0.92*thetad3 - 1.84*thetad1*cos(theta5)^2 - 1.84*thetad2*cos(theta5)^2 - 1.84*thetad3*cos(theta5)^2 + 0.49*thetad4*cos(theta5) + 0.98*thetad5*cos(theta5) + 0.835*thetad4*sin(theta5) + 1.67*thetad5*sin(theta5) + 1.17*thetad1*cos(theta5)*sin(theta5) + 1.17*thetad2*cos(theta5)*sin(theta5) + 1.17*thetad3*cos(theta5)*sin(theta5) ;
C(4,1) = 0.89445*thetad1*cos(theta4) + 0.89445*thetad2*cos(theta4) + 0.447225*thetad3*cos(theta4) + 0.49*thetad5*cos(theta5) - 0.4836*thetad1*sin(theta4) - 0.4836*thetad2*sin(theta4) - 0.2418*thetad3*sin(theta4) + 0.835*thetad5*sin(theta5) + 0.89445*thetad1*cos(theta3)*cos(theta4) + 0.447225*thetad2*cos(theta3)*cos(theta4) + 0.000825*thetad3*cos(theta3)*cos(theta4) - 0.4836*thetad1*cos(theta3)*sin(theta4) - 0.4836*thetad1*cos(theta4)*sin(theta3) - 0.2418*thetad2*cos(theta3)*sin(theta4) - 0.2418*thetad2*cos(theta4)*sin(theta3) - 0.2418*thetad3*cos(theta3)*sin(theta4) - 0.2418*thetad3*cos(theta4)*sin(theta3) - 0.89445*thetad1*sin(theta3)*sin(theta4) - 0.447225*thetad2*sin(theta3)*sin(theta4) - 0.000825*thetad3*sin(theta3)*sin(theta4) ;
C(4,2) = 0.89445*thetad1*cos(theta4) + 0.89445*thetad2*cos(theta4) + 0.447225*thetad3*cos(theta4) + 0.49*thetad5*cos(theta5) - 0.4836*thetad1*sin(theta4) - 0.4836*thetad2*sin(theta4) - 0.2418*thetad3*sin(theta4) + 0.835*thetad5*sin(theta5) + 0.447225*thetad1*cos(theta3)*cos(theta4) - 0.2418*thetad1*cos(theta3)*sin(theta4) - 0.2418*thetad1*cos(theta4)*sin(theta3) - 0.447225*thetad1*sin(theta3)*sin(theta4) ;
C(4,3) = 0.447225*thetad1*cos(theta4) + 0.447225*thetad2*cos(theta4) + 0.49*thetad5*cos(theta5) - 0.2418*thetad1*sin(theta4) - 0.2418*thetad2*sin(theta4) + 0.835*thetad5*sin(theta5) + 0.000825*thetad1*cos(theta3)*cos(theta4) - 0.2418*thetad1*cos(theta3)*sin(theta4) - 0.2418*thetad1*cos(theta4)*sin(theta3) - 0.000825*thetad1*sin(theta3)*sin(theta4) ;
C(4,4) = 0.0 ;
C(4,5) = 0.49*thetad1*cos(theta5) + 0.49*thetad2*cos(theta5) + 0.49*thetad3*cos(theta5) + 0.835*thetad1*sin(theta5) + 0.835*thetad2*sin(theta5) + 0.835*thetad3*sin(theta5) ;
C(5,1) = 1.84*thetad1*cos(theta5)^2 - 0.92*thetad2 - 0.92*thetad3 - 0.92*thetad1 + 1.84*thetad2*cos(theta5)^2 + 1.84*thetad3*cos(theta5)^2 - 0.49*thetad4*cos(theta5) - 0.835*thetad4*sin(theta5) - 1.17*thetad1*cos(theta5)*sin(theta5) - 1.17*thetad2*cos(theta5)*sin(theta5) - 1.17*thetad3*cos(theta5)*sin(theta5) ;
C(5,2) = 1.84*thetad1*cos(theta5)^2 - 0.92*thetad2 - 0.92*thetad3 - 0.92*thetad1 + 1.84*thetad2*cos(theta5)^2 + 1.84*thetad3*cos(theta5)^2 - 0.49*thetad4*cos(theta5) - 0.835*thetad4*sin(theta5) - 1.17*thetad1*cos(theta5)*sin(theta5) - 1.17*thetad2*cos(theta5)*sin(theta5) - 1.17*thetad3*cos(theta5)*sin(theta5) ;
C(5,3) = 1.84*thetad1*cos(theta5)^2 - 0.92*thetad2 - 0.92*thetad3 - 0.92*thetad1 + 1.84*thetad2*cos(theta5)^2 + 1.84*thetad3*cos(theta5)^2 - 0.49*thetad4*cos(theta5) - 0.835*thetad4*sin(theta5) - 1.17*thetad1*cos(theta5)*sin(theta5) - 1.17*thetad2*cos(theta5)*sin(theta5) - 1.17*thetad3*cos(theta5)*sin(theta5) ;
C(5,4) = - 0.49*thetad1*cos(theta5) - 0.49*thetad2*cos(theta5) - 0.49*thetad3*cos(theta5) - 0.835*thetad1*sin(theta5) - 0.835*thetad2*sin(theta5) - 0.835*thetad3*sin(theta5) ;
C(5,5) = 0.0 ;



G=zeros(5,1);
G(1) = 0.0 ;
G(2) = 19.118709000000000552432766198763*cos(theta2) - 3.9141900000000005022116056352388*sin(theta2) + 11.582667*cos(theta2)*cos(theta3) - 6.897411*cos(theta2)*sin(theta3) - 6.897411*cos(theta3)*sin(theta2) - 11.582667*sin(theta2)*sin(theta3) + 9.488232*cos(theta2)*sin(theta3)*sin(theta4) + 9.488232*cos(theta3)*sin(theta2)*sin(theta4) + 9.488232*cos(theta4)*sin(theta2)*sin(theta3) + 17.549109*sin(theta2)*sin(theta3)*sin(theta4) - 9.488232*cos(theta2)*cos(theta3)*cos(theta4) - 17.549109*cos(theta2)*cos(theta3)*sin(theta4) - 17.549109*cos(theta2)*cos(theta4)*sin(theta3) - 17.549109*cos(theta3)*cos(theta4)*sin(theta2) ;
G(3) = 11.582667*cos(theta2)*cos(theta3) - 6.897411*cos(theta2)*sin(theta3) - 6.897411*cos(theta3)*sin(theta2) - 11.582667*sin(theta2)*sin(theta3) + 9.488232*cos(theta2)*sin(theta3)*sin(theta4) + 9.488232*cos(theta3)*sin(theta2)*sin(theta4) + 9.488232*cos(theta4)*sin(theta2)*sin(theta3) + 17.549109*sin(theta2)*sin(theta3)*sin(theta4) - 9.488232*cos(theta2)*cos(theta3)*cos(theta4) - 17.549109*cos(theta2)*cos(theta3)*sin(theta4) - 17.549109*cos(theta2)*cos(theta4)*sin(theta3) - 17.549109*cos(theta3)*cos(theta4)*sin(theta2) ;
G(4) = 9.488232*cos(theta2)*sin(theta3)*sin(theta4) + 9.488232*cos(theta3)*sin(theta2)*sin(theta4) + 9.488232*cos(theta4)*sin(theta2)*sin(theta3) + 17.549109*sin(theta2)*sin(theta3)*sin(theta4) - 9.488232*cos(theta2)*cos(theta3)*cos(theta4) - 17.549109*cos(theta2)*cos(theta3)*sin(theta4) - 17.549109*cos(theta2)*cos(theta4)*sin(theta3) - 17.549109*cos(theta3)*cos(theta4)*sin(theta2) ;
G(5) = 0.0 ;






thetadd = pinv(M) * (tau - C*td-G);


return

== matlab function Dyn_Nonlinear_Forcefour/MATLAB Function3 ==
  data: J output; t input
function J  = fcn(t)
theta1 = t(1); theta2 = t(2); theta3 = t(3); 
theta4 = t(4); theta5 = t(5); 


T01 = [cos(theta1),0,sin(theta1),0;sin(theta1),0,-cos(theta1),0;0,1,0,0;0,0,0,1];
T12 = [cos(theta2),-sin(theta2),0,0.50*cos(theta2);sin(theta2),cos(theta2),0,0.50*sin(theta2);0,0,1,0;0,0,0,1];
T23 = [cos(theta3),-sin(theta3),0,0.50*cos(theta3);sin(theta3),cos(theta3),0,0.50*sin(theta3);0,0,1,0;0,0,0,1];
T34 = [cos(theta4),0,-sin(theta4),0;sin(theta4),0,cos(theta4),0;0,-1,0,0;0,0,0,1];
T45 = [cos(theta5),-sin(theta5),0,0;sin(theta5),cos(theta5),0,0;0,0,1,0.15;0,0,0,1];

T02 = T01 * T12 ;
T03 = T01 * T12 * T23 ; 
T04 = T01 * T12 * T23 * T34 ;
T0e=  T01 * T12 * T23 * T34 * T45 ;

z1 = T01(1:3, 3);
z2 = T02(1:3, 3);
z3 = T03(1:3, 3);
z4 = T04(1:3, 3);
z5 = T0e(1:3, 3);

o1 = T01(1:3, 4);
o2 = T02(1:3, 4);
o3 = T03(1:3, 4);
o4 = T04(1:3, 4);
o5 = T0e(1:3, 4);

J1 = [cross(z1, (o5 - o1))];
J2 = [cross(z2, (o5 - o2))];
J3 = [cross(z3, (o5 - o3))];
J4 = [cross(z4, (o5 - o4))];
J5 = [cross(z5, (o5 - o5))];
J_alternative_V = [J1 J2 J3 J4 J5];


J=J_alternative_V;
return;

== matlab function Dyn_Nonlinear_Forcefour/MATLAB Function4 ==
  data: ax input; dt input; ateta output; J input; dJ input
function ateta= fcn(ax,dt,J,dJ)
 Jt=pinv(J);
 
 ateta=Jt*(ax-dJ*dt);

return;

== matlab function Dyn_Nonlinear_Forcefour/MATLAB Function5 ==
  data: t input; X output
function X = fcn(t)
theta1 = t(1); theta2 = t(2); theta3 = t(3); 
theta4 = t(4); theta5 = t(5); 


T01 = [cos(theta1),0,sin(theta1),0;sin(theta1),0,-cos(theta1),0;0,1,0,0;0,0,0,1];
T12 = [cos(theta2),-sin(theta2),0,0.50*cos(theta2);sin(theta2),cos(theta2),0,0.50*sin(theta2);0,0,1,0;0,0,0,1];
T23 = [cos(theta3),-sin(theta3),0,0.50*cos(theta3);sin(theta3),cos(theta3),0,0.50*sin(theta3);0,0,1,0;0,0,0,1];
T34 = [cos(theta4),0,-sin(theta4),0;sin(theta4),0,cos(theta4),0;0,-1,0,0;0,0,0,1];
T45 = [cos(theta5),-sin(theta5),0,0;sin(theta5),cos(theta5),0,0;0,0,1,0.15;0,0,0,1];

T02 = T01 * T12 ;
T03 = T01 * T12 * T23 ; 
T04 = T01 * T12 * T23 * T34 ;
T0e=  T01 * T12 * T23 * T34 * T45 ;


X=T0e(1:3,4);

return;

== matlab function Dyn_Nonlinear_Forcefour/MATLAB Function6 ==
  data: deltaf input; ax output; X_dot input
function ax = fcn(deltaf,X_dot)
Bc = 20 ; Mc = 15 ;
ax = -Bc/Mc * X_dot + 1/Mc * deltaf ; 


return;
